simulink model "zero_if_rx"  (R2021b)
settings: Solver=VariableStepAuto  StartTime=0.0  StopTime=0.05  RelTol=1e-3
libraries: dsparch4 x3
settings Model: Creator=EternoPax  LastModifiedBy=EternoPax

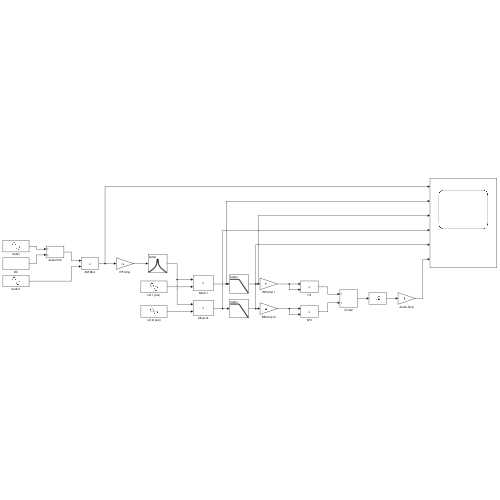
[thumbnail: Simulink's stored preview of the top-level diagram]
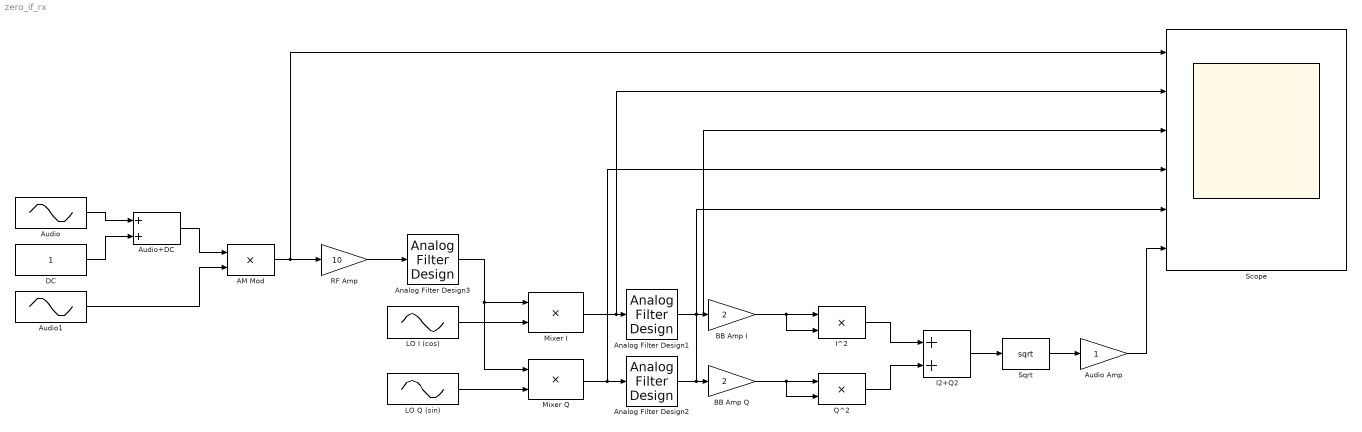
== system zero_if_rx ==
  AM Mod : Product
  Analog Filter Design1 : dsparch4/Analog Filter Design  method=Butterworth  filttype=Lowpass  N=8  Wlo=2000  Whi=80  Rp=2  Rs=40
  Analog Filter Design2 : dsparch4/Analog Filter Design  method=Butterworth  filttype=Lowpass  N=8  Wlo=2000  Whi=80  Rp=2  Rs=40
  Analog Filter Design3 : dsparch4/Analog Filter Design  method=Butterworth  filttype=Bandpass  N=8  Wlo=998000  Whi=1002000  Rp=2  Rs=40
  Audio : Sin  Amplitude=0.8  Frequency=1000  SampleTime=0
  Audio Amp : Gain
  Audio+DC : Sum
  Audio1 : Sin  Amplitude=0.8  Frequency=1000000  SampleTime=0
  BB Amp I : Gain  Gain=2
  BB Amp Q : Gain  Gain=2
  DC : Constant
  I2+Q2 : Sum
  I^2 : Product
  LO I (cos) : Sin  Frequency=1000000  SampleTime=0
  LO Q (sin) : Sin  Frequency=1000000  Phase=-90  SampleTime=0
  Mixer I : Product
  Mixer Q : Product
  Q^2 : Product
  RF Amp : Gain  Gain=10
  Scope : Scope  NumInputPorts=6
  Sqrt : Sqrt  SaturateOnIntegerOverflow=on
  wires:
  Audio/1 -> Audio+DC/1
  DC/1 -> Audio+DC/2
  Audio+DC/1 -> AM Mod/1
  Audio1/1 -> AM Mod/2
  RF Amp/1 -> Analog Filter Design3/1
  LO Q (sin)/1 -> Mixer Q/2
  Mixer I/1 -> Scope/2, Analog Filter Design1/1
  Mixer Q/1 -> Scope/4, Analog Filter Design2/1
  Analog Filter Design1/1 -> Scope/3, BB Amp I/1
  Analog Filter Design2/1 -> Scope/5, BB Amp Q/1
  BB Amp I/1 -> I^2/2, I^2/1
  BB Amp Q/1 -> Q^2/2, Q^2/1
  I^2/1 -> I2+Q2/1
  Q^2/1 -> I2+Q2/2
  I2+Q2/1 -> Sqrt/1
  Sqrt/1 -> Audio Amp/1
  AM Mod/1 -> Scope/1, RF Amp/1
  Analog Filter Design3/1 -> Mixer Q/1, Mixer I/1
  LO I (cos)/1 -> Mixer I/2
  Audio Amp/1 -> Scope/6
